simulink model "ModeloFinal_peliedit"  (Simulink 8.7)
settings: Solver=ode4  StartTime=0.0  StopTime=20  FixedStep=0.001  RelTol=1e-3
values from neighbouring files (symbols this model uses):
  Ke = 0.00767    [dynamic_script.m]
  Kt = 0.00767    [dynamic_script.m]
  La = 0.18    [dynamic_script.m]
  Ra = 2.6    [dynamic_script.m]
  Vin = 0    [dynamic_script.m]
undefined symbols (not defined in the file or in its folder): Kr, theta_ini, thetadot_ini
settings Model: Creator=User PC  LastModifiedBy=gabri
settings DebuggingCC: UnderspecifiedInitializationDetection=Simplified  MergeDetectMultiDrivingBlocksExec=error

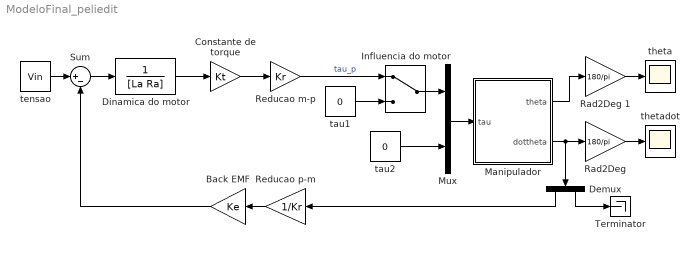
== system ModeloFinal_peliedit ==
  Back EMF : Gain  Gain=Ke
  Constante de torque : Gain  Gain=Kt
  Demux : Demux  Outputs=2
  Dinamica do motor : TransferFcn  Denominator=[La Ra]
  Influencia do motor : ManualSwitch
  Manipulador : Subsystem
  Mux : Mux  Inputs=2
  "Rad2Deg " : Gain  Gain=180/pi
  Rad2Deg 1 : Gain  Gain=180/pi
  Reducao m-p : Gain  Gain=Kr
  Reducao p-m : Gain  Gain=1/Kr
  Sum : Sum  Inputs=|+-
  Terminator : Terminator
  tau1 : Constant  Value=0
  tau2 : Constant  Value=0
  tensao : Constant  Value=Vin
  "theta " : Scope
  thetadot : Scope
  wires:
  Sum/1 -> Dinamica do motor/1
  Dinamica do motor/1 -> Constante de torque/1
  Constante de torque/1 -> Reducao m-p/1
  Reducao p-m/1 -> Back EMF/1
  Back EMF/1 -> Sum/2
  tensao/1 -> Sum/1
  Reducao m-p/1 -> Influencia do motor/1  "tau_p"
  tau2/1 -> Mux/2
  Demux/2 -> Terminator/1
  Rad2Deg 1/1 -> "theta "/1
  Demux/1 -> Reducao p-m/1
  "Rad2Deg "/1 -> thetadot/1
  tau1/1 -> Influencia do motor/2
  Influencia do motor/1 -> Mux/1
  Manipulador/2(dottheta) -> Demux/1, "Rad2Deg "/1
  Mux/1 -> Manipulador/1(tau)
  Manipulador/1(theta) -> Rad2Deg 1/1

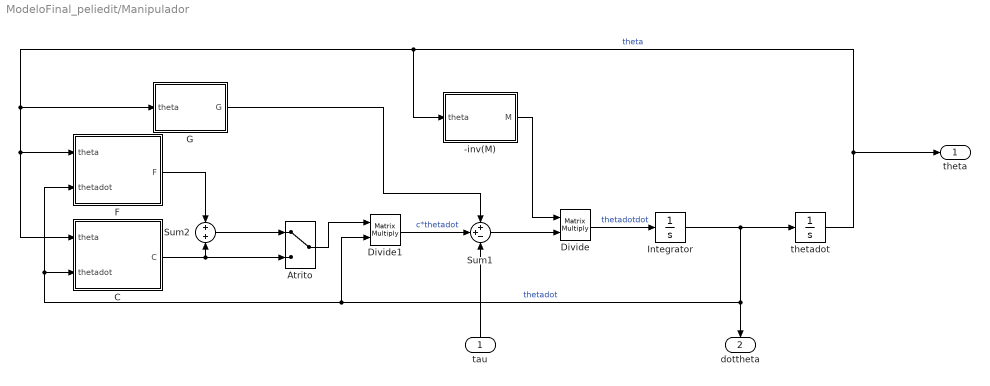
== system ModeloFinal_peliedit/Manipulador ==
  tau : Inport
  -inv(M) : MATLAB Function  TreatAsAtomicUnit=on
  Atrito : ManualSwitch
  C : MATLAB Function  TreatAsAtomicUnit=on
  Divide : Product  Inputs=**  Multiplication=Matrix(*)
  Divide1 : Product  Inputs=**  Multiplication=Matrix(*)
  F : MATLAB Function  TreatAsAtomicUnit=on
  G : MATLAB Function  TreatAsAtomicUnit=on
  Integrator : Integrator  InitialCondition=thetadot_ini
  Sum1 : Sum  Inputs=++-
  Sum2 : Sum  Inputs=+|+
  thetadot : Integrator  InitialCondition=theta_ini
  theta : Outport
  dottheta : Outport  Port=2
  wires:
  G/1(G) -> Sum1/1
  -inv(M)/1(M) -> Divide/1
  C/1(C) -> Atrito/2, Sum2/2
  Sum1/1 -> Divide/2
  Divide1/1 -> Sum1/2  "c*thetadot"
  Divide/1 -> Integrator/1  "thetadotdot"
  tau/1 -> Sum1/3
  Atrito/1 -> Divide1/1
  Sum2/1 -> Atrito/1
  thetadot/1 -> theta/1, -inv(M)/1(theta), F/1(theta), C/1(theta), G/1(theta)  "theta"
  F/1(F) -> Sum2/1
  Integrator/1 -> F/2(thetadot), C/2(thetadot), Divide1/2, dottheta/1, thetadot/1  "thetadot"

== matlab function Manipulador/-inv(M) ==
  data: theta input double; M output double
function M = fcn(theta)
m1 = 0.25;
l1 = 0.187;
w1 = 0.038;
m2 = 0.15;
l2 = 0.34;
r = 0.0065;
g = 9.8;
Kr = 70;

Je = 2.8e-6 + 2.27e-5 + 5e-7;
Jm = 3.87e-7;

M = [(m1/12)*(w1^2+l1^2)+m1*(l1/2)^2+m2*(l1^2)+m2*(l2/2)^2*(sin(theta(2,1)))^2+m2/12*(3*r^2+l2^2*(sin(theta(2,1)))^2+3*(r^2)*(cos(theta(2,1)))^2),...
    -0.5*m2*l1*l2*cos(theta(2,1));...
    -0.5*m2*l1*l2*cos(theta(2,1)),...
    (1/12)*m2*(3*r^2+l2^2)+m2*(l2/2)^2 ];

M_motor = [Je+(Kr^2)*Jm, 0; 0, 0];

M = M + M_motor;  % inercia do motor

M = -inv(M);

== matlab function Manipulador/C ==
  data: theta input double; C output double; thetadot input double
function C = fcn(theta,thetadot)
m1 = 0.25;
l1 = 0.187;
w1 = 0.038;
m2 = 0.15;
l2 = 0.34;
r = 0.0065;
g = 9.8;
%#codegen
C = [0 ...
    ((m2*sin(2*theta(2,1))*((l2^2)/3 -(r^2)/4))*thetadot(1,1))+(0.5*m2*l1*l2*sin(theta(2,1))*thetadot(2,1));...
    (-(m2*sin(2*theta(2,1))*((l2^2)/3 -(r^2)/4))*thetadot(1,1))-(0.25*m2*l1*l2*sin(theta(2,1))*thetadot(2,1))...
    (0.25*m2*l1*l2*sin(theta(2,1))*thetadot(1,1))];

== matlab function Manipulador/G ==
  data: theta input double; G output double
function G = fcn(theta)
%#codegen
m1 = 0.25;
l1 = 0.187;
w1 = 0.038;
m2 = 0.15;
l2 = 0.34;
r = 0.0065;
g = 9.8;

G=[0; -m2*g*l2*sin(theta(2,1))*0.5];

== matlab function Manipulador/F ==
  data: theta input double; F output double; thetadot input double
function F = fcn(theta,thetadot)
m1 = 0.25;
l1 = 0.187;
w1 = 0.038;
m2 = 0.15;
l2 = 0.34;
r = 0.0065;
g = 9.8;

F = [2e-3, 0;...
     0   , 7e-4];
